simulink model "Sim"  (R2025b)
settings: Solver=VariableStepAuto  StartTime=0.0  StopTime=100  RelTol=1e-3
values from neighbouring files (symbols this model uses):
  hiddenLayerSizeCtrl = (2 * inputLayerSizeCtrl + 1) * 1    (= 13)    [Init.m]
  n = 4    [Init.m]
  p = 2    [Init.m]
  u_max = 12 * [1; 0.8]    [Init.m]
  u_min = - 12 * [1; 0.8]    [Init.m]
  Vctrl0 = 0.1 * randn(hiddenLayerSizeCtrl, inputLayerSizeCtrl)    [Init.m]
  Wctrl0 = 0.1 * randn(outputLayerSizeCtrl, hiddenLayerSizeCtrl)    [Init.m]
  x0 = [0; 0.5; 0.1; 0]    [Init.m]
settings Model: Creator=Asus  LastModifiedBy=Asus

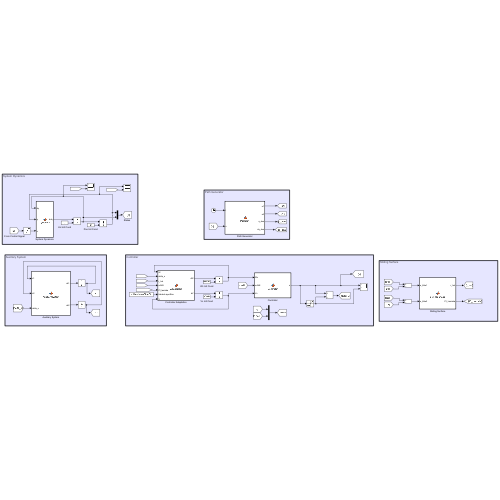
[thumbnail: Simulink's stored preview of the top-level diagram]
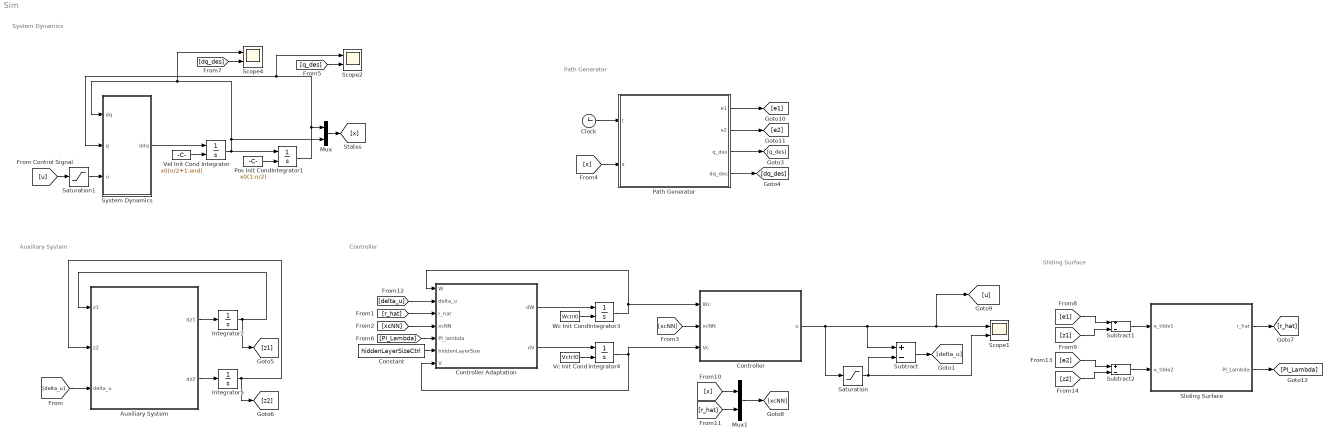
== system Sim ==
  note: System Dynamics
  note: Path Generator
  note: Auxiliary System
  note: Controller
  note: Sliding Surface
  Auxiliary System : MATLAB Function  TreatAsAtomicUnit=on
  Clock : Clock
  Constant : Constant  Value=hiddenLayerSizeCtrl
  Controller : MATLAB Function  TreatAsAtomicUnit=on
  Controller Adaptation : MATLAB Function  TreatAsAtomicUnit=on
  Integrator{,1,3..4} (4 alike) : Integrator  InitialConditionSource=external  InitialCondition=[0.5; 0.5]
  Integrator2 : Integrator  InitialCondition=zeros(p, 1)
  Integrator5 : Integrator  InitialCondition=zeros(p, 1)
  Mux : Mux  Inputs=2
  Mux1 : Mux  Inputs=2
  Path Generator : MATLAB Function  TreatAsAtomicUnit=on
  Pos Init Cond : Constant  Value=x0(1:n/2)
  Saturation : Saturate  UpperLimit=u_max  LowerLimit=u_min
  Saturation1 : Saturate  UpperLimit=u_max  LowerLimit=u_min
  Scope1 : Scope  NumInputPorts=2
      settings: ActiveDisplayYMinimum=-13.35514879633242  ActiveDisplayYMaximum=31.546961195274957
  Scope2 : Scope  NumInputPorts=2
      settings: ActiveDisplayYMinimum=-1.16864  ActiveDisplayYMaximum=0.77004
  Scope4 : Scope  NumInputPorts=2
      settings: ActiveDisplayYMinimum=-3.08844  ActiveDisplayYMaximum=2.66268  DataLoggingVariableName=ScopeData3
  Sliding Surface : MATLAB Function  TreatAsAtomicUnit=on
  Subtract : Sum  Inputs=+-
  Subtract1 : Sum  Inputs=+-
  Subtract2 : Sum  Inputs=+-
  System Dynamics : MATLAB Function  TreatAsAtomicUnit=on
  Vc Init Cond : Constant  Value=Vctrl0
  Vel Init Cond : Constant  Value=x0(n/2+1:end)
  Wc Init Cond : Constant  Value=Wctrl0
  wires:
  [u] -> Saturation1/1
  System Dynamics/1(ddq) -> Integrator/1
  Vel Init Cond/1 -> Integrator/2
  Pos Init Cond/1 -> Integrator1/2
  Integrator/1 -> Integrator1/1, Mux/2, Scope4/1, System Dynamics/1(dq)
  Mux/1 -> [x]
  Integrator1/1 -> Scope2/1, System Dynamics/2(q), Mux/1
  Clock/1 -> Path Generator/1(t)
  Auxiliary System/1(dz1) -> Integrator2/1
  Integrator2/1 -> [z1], Auxiliary System/1(z1)
  [delta_u] -> Auxiliary System/3(delta_u)
  Controller/1(u) -> Saturation/1, Subtract/1, [u], Scope1/1
  Wc Init Cond/1 -> Integrator3/2
  Controller Adaptation/1(dW) -> Integrator3/1
  Integrator3/1 -> Controller/1(Wc), Controller Adaptation/1(W)
  Controller Adaptation/2(dV) -> Integrator4/1
  Vc Init Cond/1 -> Integrator4/2
  Integrator4/1 -> Controller Adaptation/7(V), Controller/3(Vc)
  [r_hat] -> Controller Adaptation/3(r_hat)
  [xcNN] -> Controller Adaptation/4(xcNN)
  [xcNN] -> Controller/2(xcNN)
  Auxiliary System/2(dz2) -> Integrator5/1
  Integrator5/1 -> [z2], Auxiliary System/2(z2)
  [x] -> Path Generator/2(x)
  Mux1/1 -> [xcNN]
  [r_hat] -> Mux1/2
  [x] -> Mux1/1
  Saturation/1 -> Scope1/2, Subtract/2
  Subtract/1 -> [delta_u]
  [delta_u] -> Controller Adaptation/2(delta_u)
  Constant/1 -> Controller Adaptation/6(hiddenLayerSize)
  Sliding Surface/1(r_hat) -> [r_hat]
  [e1] -> Subtract1/1
  [z1] -> Subtract1/2
  Subtract1/1 -> Sliding Surface/1(e_tilde1)
  [z2] -> Subtract2/2
  [e2] -> Subtract2/1
  Subtract2/1 -> Sliding Surface/2(e_tilde2)
  Path Generator/2(e2) -> [e2]
  Path Generator/1(e1) -> [e1]
  Path Generator/4(dq_des) -> [dq_des]
  Path Generator/3(q_des) -> [q_des]
  [q_des] -> Scope2/2
  [PI_Lambda] -> Controller Adaptation/5(PI_lambda)
  Sliding Surface/2(PI_Lambda) -> [PI_Lambda]
  [dq_des] -> Scope4/2
  Saturation1/1 -> System Dynamics/3(u)

== matlab function Sim/Auxiliary System ==
  data: z1 input; z2 input; dz1 output; delta_u input; dz2 output
function [dz1, dz2] = AuxiliarySystem(z1, z2, delta_u)
    
    K1  = 5 * diag([-1, -1]); K2  = 5 * diag([-1, -1]);
    h1  = 5 * [-1; -1]; h2  = 5 * [-1; -1];

    dz1 = K1 * z1 + h1 * delta_u(1);
    dz2 = K2 * z2 + h2 * delta_u(2);
    
end

== matlab function Sim/System Dynamics ==
  data: dq input; q input; ddq output; u input
function ddq = Dynamics(dq, q, u)

    % Robot Params
    m1 = 1;                 % mass of link 1
    m2 = 1;                 % mass of link 2
    l1 = 0.5;               % length of link 1
    lc1 = l1/2;             % length of center of mass link 1 
    l2 = 0.5;               % length of link 2
    lc2 = l2/2;             % length of center of mass link 2
    I1 = 1/12 * m1 * l1^2;  % inertia moment link 1
    I2 = 1/12 * m2 * l2^2;  % inertia moment link 2
    gravity = 9.81;         % gravity constant

    % M(q) Matrix
    M11 = m1 * lc1^2 + I1 + m2 * (l1^2 + ...
        lc2^2 + 2 * l1 * lc2 * cos(q(2))) + I2;
    M12 = m2 * l1 * lc2 *cos(q(2)) + m2 * lc2^2 + I2;
    M21 = M12;
    M22 = m2 * lc2^2 + I2;
    M = [M11 M12; M21 M22];
     
    % G(q) Vector
    G1 = m1 * lc1 * gravity * cos(q(1)) + m2 * gravity * ...
        (lc2 * cos(q(1) + q(2)) + l1 * cos(q(1)));
    G2 = m2 * lc2 * gravity * cos(q(1) + q(2));
    G = [G1; G2];
    
    % C(q,qdot) Matrix
    h = m2 * l1 * lc2 * sin(q(2));
    C = [-h * dq(2), -h * (dq(1) + dq(2)); h * dq(1), 0];
    
    % robot dynamics
    ddq = M \ (u - C * dq - G);
    y   = q;
    psi = ddq;

end

== matlab function Sim/Path Generator ==
  data: t input; x input; e1 output; e2 output; q_des output; dq_des output
function [e1, e2, q_des, dq_des] = PathGen(t, x)
    
    w = 0.2;
    A = 0.5;

    q_des   = A *       [ sin(w*t);  cos(w*t)];
    dq_des  = A * w *   [ cos(w*t); -sin(w*t)];
    % ddq_des = A * w^2 * [-sin(w*t); -cos(w*t)];

    y_bar1 = x([1, 3]); y_bar2 = x([2, 4]);

    y_bar_des1 = [q_des(1); dq_des(1)];
    y_bar_des2 = [q_des(2); dq_des(2)];

    e1 = y_bar1 - y_bar_des1;
    e2 = y_bar2 - y_bar_des2;
    
end

== matlab function Sim/Controller ==
  data: u output; Wc input; xcNN input; Vc input
function u = Controller(Wc, xcNN, Vc)

    Sigma = @(z) (-1 + 2 ./ (1 + exp(-2 * z)));

    u = - Wc * Sigma(Vc * xcNN);
    
end

== matlab function Sim/Controller Adaptation ==
  data: dW output; dV output; W input; delta_u input; r_hat input; xcNN input; PI_lambda input; hiddenLayerSize input; V input
function [dW, dV] = Adaptation(W, delta_u, r_hat, xcNN, PI_lambda, hiddenLayerSize, V)
    
    Sigma = @(z) (-1 + 2 ./ (1 + exp(-2 * z)));

    Ac1 = [0, 1; -1, -2]; B1 = [0; 1];
    Ac2 = [0, 1; -1, -2]; B2 = [0; 1];
    
    Ac = blkdiag(Ac1, Ac2);
    B  = blkdiag(B1, B2);

    K1 = 5 * diag([-1, -1]); K2  = 5 * diag([-1, -1]);
    K  = blkdiag(K1, K2);

    h1 = 5 * [-1; -1]; h2  = 5 * [-1; -1];
    h  = blkdiag(h1, h2); % bug potential

    eta   = [1, 1];
    gamma = [0.001, 0.001];

    PI_c = diag(Sigma(V * xcNN).^2);
    
    dW = eta(1) * (r_hat' * PI_lambda * (-Ac^(-1) * B + K^(-1) * h * delta_u))' * Sigma(V * xcNN)' - gamma(1) * norm(r_hat) * W;
    dV = eta(2) * (r_hat' * PI_lambda * (-Ac^(-1) * B + K^(-1) * h * delta_u) * W * (eye(hiddenLayerSize) - PI_c))' * tanh(xcNN') - gamma(2) * norm(r_hat) * V;

end

== matlab function Sim/Sliding Surface ==
  data: e_tilde1 input; r_hat output; e_tilde2 input; PI_Lambda output
function [r_hat, PI_Lambda] = SlidingSurface(e_tilde1, e_tilde2)

    Lambda1 = 5; Lambda2 = 5;

    r_hat1  = [Lambda1, 1] * e_tilde1;
    r_hat2  = [Lambda2, 1] * e_tilde2;

    r_hat   = [r_hat1; r_hat2];

    PI_Lambda = blkdiag([Lambda1, 1], [Lambda2, 1]);
    
end
